simulink model "Main"  (R2024a)
settings: Solver=VariableStepAuto  StartTime=0.0  StopTime=100  RelTol=1e-7
values from neighbouring files (symbols this model uses):
  A = [0 1; -g/l -b/(m*l)]    [BasaleDynamicaSym.m]
  amp = 1    [BasaleDynamicaSym.m]
  B = [0; 1/(m*l)]    [BasaleDynamicaSym.m]
  b = 1.2    [BasaleDynamicaSym.m]    (also in dampingcoefficientscript.m)
  C = [1 0]    [BasaleDynamicaSym.m]
  d = [0; -(amp*freq)/l]    [BasaleDynamicaSym.m]
  freq = 1    [BasaleDynamicaSym.m]
  g = 9.81    [BasaleDynamicaSym.m]    (also in dampingcoefficientscript.m)
  H = (freq^2)/l    (= 2)    [BasaleDynamicaSym.m]
  Kf = -1/(C*inv(Ac)*B)    [BasaleDynamicaSym.m]
  l = 0.5    [BasaleDynamicaSym.m]    (also in dampingcoefficientscript.m = 0.554)
  m = 4.5    [BasaleDynamicaSym.m]    (also in dampingcoefficientscript.m)
  theta_0 = pi/4    (= 0.785398163397)    [BasaleDynamicaSym.m]    (also in dampingcoefficientscript.m = 0.349065850399)
undefined symbols (not defined in the file or in its folder): K
libraries: simulink_extras x2
settings Model: Creator=alesm  LastModifiedBy=alesm

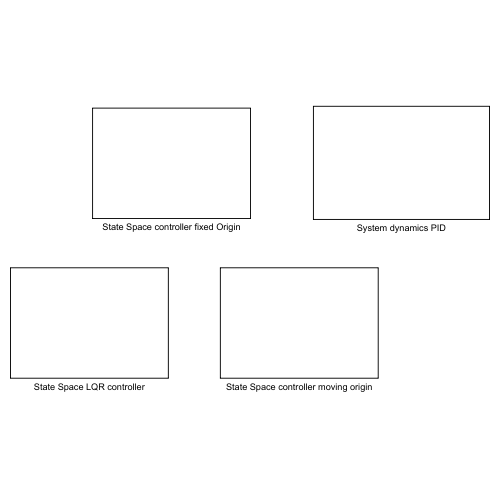
[thumbnail: Simulink's stored preview of the top-level diagram]
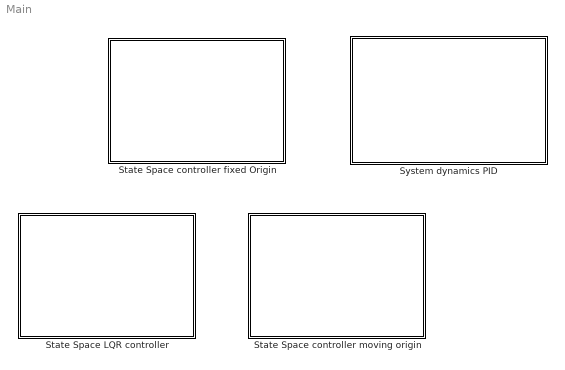
== system Main ==
  State Space LQR controller : Subsystem
  State Space controller fixed Origin : Subsystem
  State Space controller moving origin : Subsystem
  System dynamics PID : Subsystem

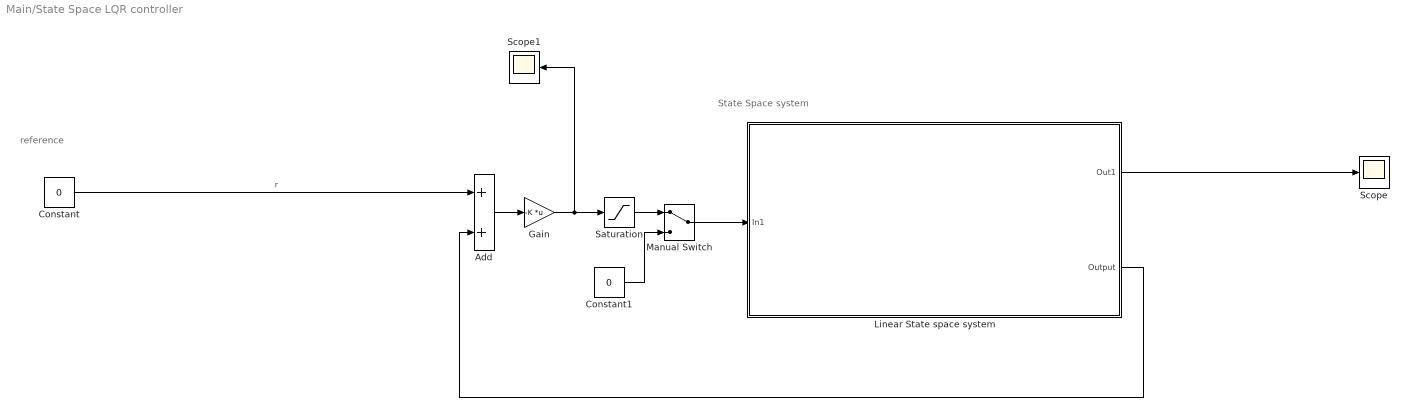
== system Main/State Space LQR controller ==
  note: reference
  note: State Space system
  Add : Sum
  Constant : Constant  Value=0
  Constant1 : Constant  Value=0
  Gain : Gain  Gain=-K  Multiplication=Matrix(K*u)
  Linear State space system : Subsystem
  Manual Switch : ManualSwitch
  Saturation : Saturate  UpperLimit=inf  LowerLimit=-inf
  Scope : Scope
  Scope1 : Scope
  wires:
  Linear State space system/1(Out1) -> Scope/1
  Constant/1 -> Add/1  "r"
  Linear State space system/2(Output) -> Add/2
  Gain/1 -> Saturation/1, Scope1/1
  Add/1 -> Gain/1
  Manual Switch/1 -> Linear State space system/1(In1)
  Constant1/1 -> Manual Switch/2
  Saturation/1 -> Manual Switch/1

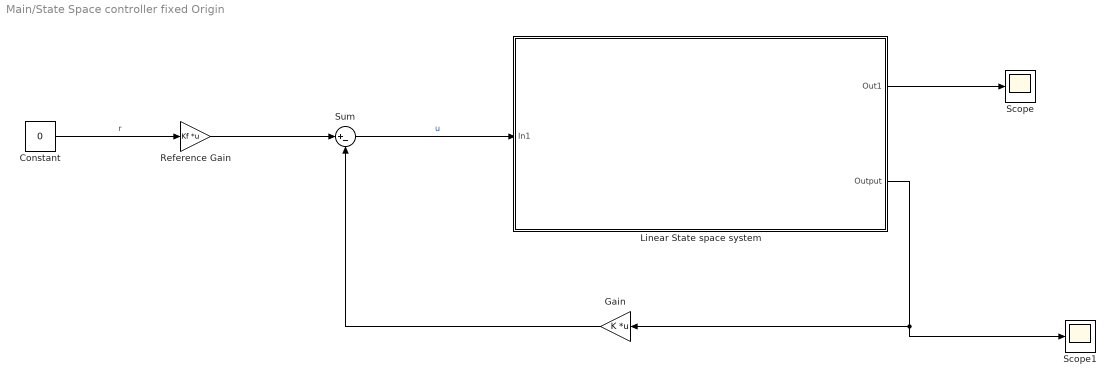
== system Main/State Space controller fixed Origin ==
  Constant : Constant  Value=0
  Gain : Gain  Gain=K  Multiplication=Matrix(K*u)
  Linear State space system : Subsystem
  Reference Gain : Gain  Gain=Kf  Multiplication=Matrix(K*u)
  Scope : Scope
  Scope1 : Scope
  Sum : Sum  Inputs=|+-
  wires:
  Sum/1 -> Linear State space system/1(In1)  "u"
  Linear State space system/2(Output) -> Scope1/1, Gain/1
  Linear State space system/1(Out1) -> Scope/1
  Gain/1 -> Sum/2
  Constant/1 -> Reference Gain/1  "r"
  Reference Gain/1 -> Sum/1

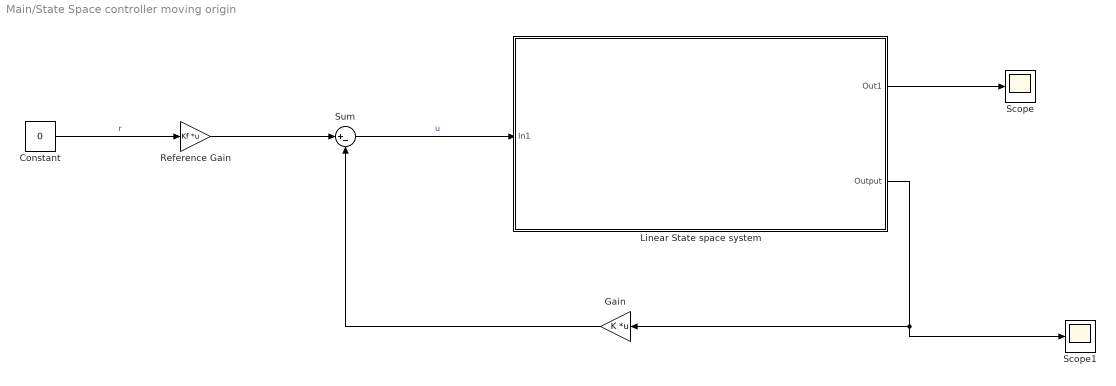
== system Main/State Space controller moving origin ==
  Constant : Constant  Value=0
  Gain : Gain  Gain=K  Multiplication=Matrix(K*u)
  Linear State space system : Subsystem
  Reference Gain : Gain  Gain=Kf  Multiplication=Matrix(K*u)
  Scope : Scope
  Scope1 : Scope
  Sum : Sum  Inputs=|+-
  wires:
  Sum/1 -> Linear State space system/1(In1)  "u"
  Linear State space system/2(Output) -> Scope1/1, Gain/1
  Linear State space system/1(Out1) -> Scope/1
  Gain/1 -> Sum/2
  Constant/1 -> Reference Gain/1  "r"
  Reference Gain/1 -> Sum/1

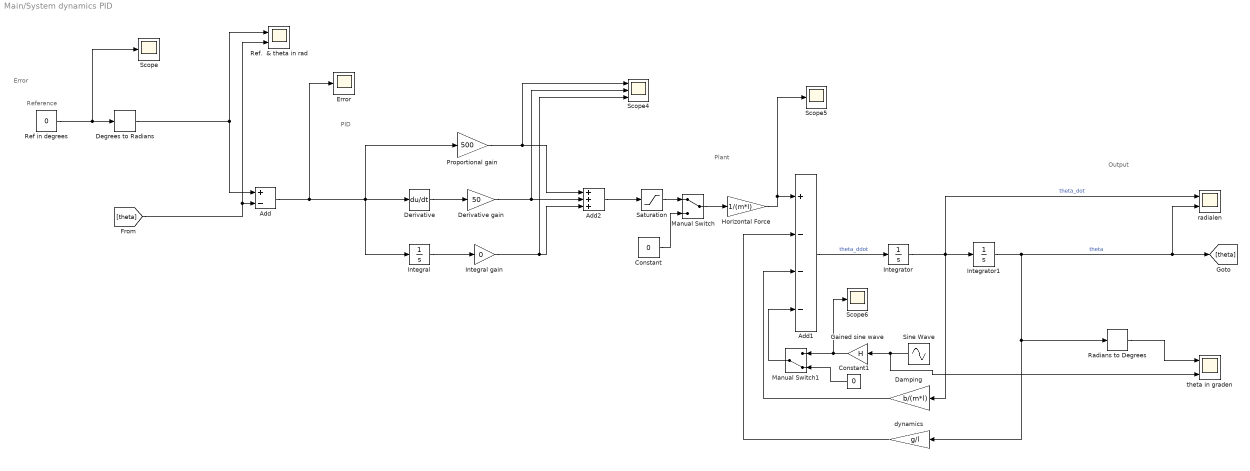
== system Main/System dynamics PID ==
  note: Output
  note: Plant
  note: Reference
  note: PID
  note: Error
  Add : Sum  Inputs=+-
  Add1 : Sum  Inputs=+---
  Add2 : Sum  Inputs=+++
  Constant : Constant  Value=0
  Constant1 : Constant  Value=0
  Damping : Gain  Gain=b/(m*l)
  Degrees to Radians : simulink_extras/Transformations/Degrees to Radians
  Derivative : Derivative
  Derivative gain : Gain  Gain=50
  Error : Scope
  Gained sine wave : Gain  Gain=H
  Horizontal Force : Gain  Gain=1/(m*l)
  Integral : Integrator
  Integral gain : Gain  Gain=0
  Integrator : Integrator
  Integrator1 : Integrator  InitialCondition=10*(pi/180)
  Manual Switch : ManualSwitch
  Manual Switch1 : ManualSwitch  CurrentSetting=0
  Proportional gain : Gain  Gain=500
  Radians to Degrees : simulink_extras/Transformations/Radians to Degrees
  Ref in degrees : Constant  Value=0  SampleTime=1
  Ref.  & theta in rad : Scope  NumInputPorts=2
  Saturation : Saturate  UpperLimit=inf  LowerLimit=-inf
  Scope : Scope
  Scope4 : Scope  NumInputPorts=3
  Scope5 : Scope
  Scope6 : Scope
  Sine Wave : Sin  Amplitude=amp  Frequency=freq  SampleTime=0
  dynamics : Gain  Gain=g/l
  radialen : Scope  NumInputPorts=2
  theta in graden : Scope  NumInputPorts=2
  wires:
  Integrator1/1 -> Radians to Degrees/1, dynamics/1, [theta], radialen/2  "theta"
  Integrator/1 -> Damping/1, Integrator1/1, radialen/1  "theta_dot"
  Degrees to Radians/1 -> Add/1, Ref.  & theta in rad/1
  [theta] -> Ref.  & theta in rad/2, Add/2
  Derivative/1 -> Derivative gain/1
  Integral/1 -> Integral gain/1
  Add1/1 -> Integrator/1  "theta_ddot"
  Horizontal Force/1 -> Scope5/1, Add1/1
  Damping/1 -> Add1/3
  dynamics/1 -> Add1/2
  Add/1 -> Error/1, Integral/1, Proportional gain/1, Derivative/1
  Derivative gain/1 -> Scope4/2, Add2/2
  Proportional gain/1 -> Scope4/1, Add2/1
  Integral gain/1 -> Scope4/3, Add2/3
  Radians to Degrees/1 -> theta in graden/1
  Sine Wave/1 -> theta in graden/2, Gained sine wave/1
  Gained sine wave/1 -> Manual Switch1/1, Scope6/1
  Ref in degrees/1 -> Scope/1, Degrees to Radians/1
  Add2/1 -> Saturation/1
  Saturation/1 -> Manual Switch/1
  Manual Switch/1 -> Horizontal Force/1
  Constant/1 -> Manual Switch/2
  Manual Switch1/1 -> Add1/4
  Constant1/1 -> Manual Switch1/2

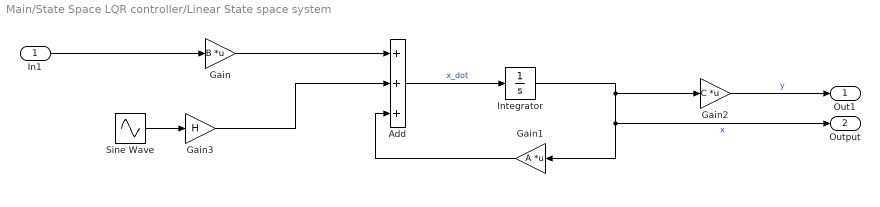
== system Main/State Space LQR controller/Linear State space system ==
  In1 : Inport
  Add : Sum  Inputs=+++
  Gain : Gain  Gain=B  Multiplication=Matrix(K*u)
  Gain1 : Gain  Gain=A  Multiplication=Matrix(K*u)
  Gain2 : Gain  Gain=C  Multiplication=Matrix(K*u)
  Gain3 : Gain  Gain=H
  Integrator : Integrator
  Sine Wave : Sin  SampleTime=0
  Out1 : Outport
  Output : Outport  Port=2
  wires:
  Integrator/1 -> Gain2/1, Gain1/1, Output/1  "x"
  Gain1/1 -> Add/3
  In1/1 -> Gain/1
  Gain2/1 -> Out1/1  "y"
  Gain/1 -> Add/1
  Sine Wave/1 -> Gain3/1
  Gain3/1 -> Add/2
  Add/1 -> Integrator/1  "x_dot"

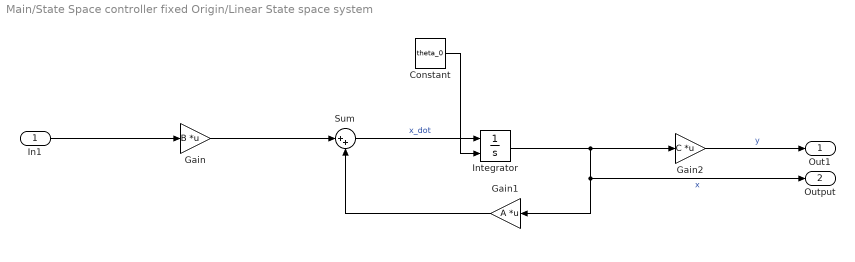
== system Main/State Space controller fixed Origin/Linear State space system ==
  In1 : Inport
  Constant : Constant  Value=theta_0
  Gain : Gain  Gain=B  Multiplication=Matrix(K*u)
  Gain1 : Gain  Gain=A  Multiplication=Matrix(K*u)
  Gain2 : Gain  Gain=C  Multiplication=Matrix(K*u)
  Integrator : Integrator  InitialConditionSource=external
  Sum : Sum  Inputs=|++
  Out1 : Outport
  Output : Outport  Port=2
  wires:
  Gain/1 -> Sum/1
  Sum/1 -> Integrator/1  "x_dot"
  Integrator/1 -> Gain2/1, Gain1/1, Output/1  "x"
  Gain1/1 -> Sum/2
  In1/1 -> Gain/1
  Gain2/1 -> Out1/1  "y"
  Constant/1 -> Integrator/2

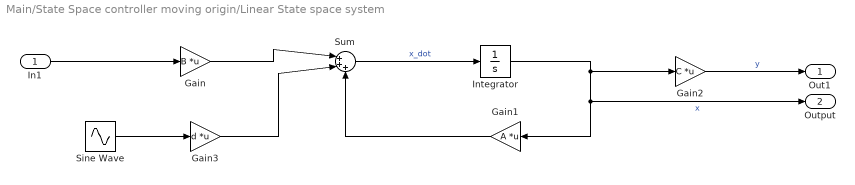
== system Main/State Space controller moving origin/Linear State space system ==
  In1 : Inport
  Gain : Gain  Gain=B  Multiplication=Matrix(K*u)
  Gain1 : Gain  Gain=A  Multiplication=Matrix(K*u)
  Gain2 : Gain  Gain=C  Multiplication=Matrix(K*u)
  Gain3 : Gain  Gain=d  Multiplication=Matrix(K*u)
  Integrator : Integrator
  Sine Wave : Sin  Amplitude=amp  Frequency=freq  SampleTime=0
  Sum : Sum  Inputs=|+++
  Out1 : Outport
  Output : Outport  Port=2
  wires:
  Gain/1 -> Sum/1
  Sum/1 -> Integrator/1  "x_dot"
  Integrator/1 -> Gain2/1, Gain1/1, Output/1  "x"
  In1/1 -> Gain/1
  Gain2/1 -> Out1/1  "y"
  Gain1/1 -> Sum/3
  Sine Wave/1 -> Gain3/1
  Gain3/1 -> Sum/2
